simulink model "torque_reflex"  (R2019b)
settings: Solver=ode4  StartTime=0.0  StopTime=inf  FixedStep=BKIN_STEP_TIME  RelTol=1e-3  EnableMultiTasking=on
StartFcn:
  |  warndlg('Dexterit-E models cannot run under simulation. Please compile your model and run it from within Dexterit-E.');set_param(bdroot,'SimulationCommand','stop')
model workspace (MAT data in the model file):
  ACTIVE = 4
  AMPLITUDE = 7
  BASE_STIFFNESS = 12
  BKIN_KINEMATIC_FRAME_SIZE = 400
  BKIN_STEP_TIME = 0.00025
  COLOR_2 = 5
  CONDITION = 3
  DELAY_POST_TRIAL = 4
  DURATION = 5
  E_END_TRIAL = 2
  E_HAND_OUT = 4
  E_NO_EVENT = 0
  E_SHOW_TARGET = 3
  E_SRS_ON = 6
  E_START_TRIAL = 5
  E_TARGET_REACHED = 1
  HAND_OUT_TIME = 6
  IMAGE = 3
  INSERT_OFFSET = 8
  L1_LENGTH = 6
  L1_LINE = 7
  L2_LENGTH = 7
  L2_LINE = 8
  LOAD = 2
  MOVE_THRESHOLD = 10
  MUSCLE = 1
  MUSCLE_LENGTH = 1
  REFLEX = 9
  REFLEX_GAIN = 5
  RESTING_FORCE = 2
  SPEED = 6
  SPRING_X = 1
  SPRING_Y = 2
  SRS_GAIN = 13
  TARGET_1 = 3
  THICKNESS = 4
  V_MAX = 3
  WALL_DAMPING = 11
  WALL_STIFFNESS = 9
  activation = 1
  col_x = 1
  col_y = 2
undefined symbols (not defined in the file or in its folder): slselsubs
libraries: Video x5, simulink x5, xpcutilitieslib x4, KINARM_IO x4, General x3, KINARM_loads x2, KINARM_EP_loads x2, KINARM_general x1, dspstat3 x1
(part 1 of 2)
settings Model: ModifiedComment=chris -- Wed Feb 16 09:18:30 2005 -- Version 1.1384  ModifiedHistory=Feb 16/05 - Add error repeat, add offset ramp  ExtModeArmWhenConnect=off  ExtModeLogAll=off  OrderedModelArguments=off  Creator=Chris Grebeldinger  LastModifiedBy=tinggroup
settings SolverCC: AutoInsertRateTranBlk=on
settings DataIOCC: SaveFormat=Array  SignalLoggingSaveFormat=ModelDataLogs  SaveOutput=off  SaveTime=off  ReturnWorkspaceOutputs=off  SignalLoggingName=sigsOut
settings OptimizationCC: BlockReduction=off  BooleanDataType=off  OptimizeBlockIOStorage=off  BufferReuse=off  GlobalBufferReuse=off  ExpressionFolding=off  ExpressionDepthLimit=2147483647  LocalBlockOutputs=off  InitFltsAndDblsToZero=on  LifeSpan=inf  OptimizeDataStoreBuffers=off  BusAssignmentInplaceUpdate=off
settings DebuggingCC: SaveWithParameterizedLinksMsg=none  UnderspecifiedInitializationDetection=Classic  MergeDetectMultiDrivingBlocksExec=none  SignalResolutionControl=TryResolveAllWithWarning  MultiTaskDSMMsg=warning  FcnCallInpInsideContextMsg=warning  BusObjectLabelMismatch=none  StateNameClashWarn=warning  StrictBusMsg=ErrorOnBusTreatedAsVector  SFUnexpectedBacktrackingDiag=warning  SFNoUnconditionalDefaultTransitionDiag=warning  SFExecutionAtInitializationDiag=none  UnderSpecifiedDimensionMsg=warning  ArithmeticOperatorsInVariantConditions=warning
settings HardwareCC: ProdBitPerPointer=32  ProdBitPerSizeT=32  ProdBitPerPtrDiffT=32  ProdLargestAtomicFloat=None  ProdWordSize=32  ProdLongLongMode=on  ProdHWDeviceType=Generic->32-bit x86 compatible  TargetHWDeviceType=32-bit Generic
settings ModelReferenceCC: PropagateSignalLabelsOutOfModel=off
settings SFSimCC: SimUseLocalCustomCode=off  SimParseCustomCode=off  CustomCodeUndefinedFunction=UseInterfaceOnly
settings RTWCC: Description=Simulink Real-Time  SystemTargetFile=slrt.tlc  TemplateMakefile=slrt_default_tmf  RTWUseLocalCustomCode=off  CustomHeaderCode=#include <stdlib.h>  CodeExecutionProfiling=on  RTWCompilerOptimization=on
settings CodeAppCC: MaxIdLength=63  StateflowObjectComments=on
settings SimulinkRealTimeCC: TargetFcnLib=ansi_tfl_tmw.mat  GeneratePreprocessorConditionals=Disable all  PreserveStateflowLocalDataDimensions=off
settings ConfigComp: CovMetricSettings=dw  CovHtmlReporting=on  CovSaveCumulativeToWorkspaceVar=on  CovSaveSingleToWorkspaceVar=on  CovExternalEMLEnable=off

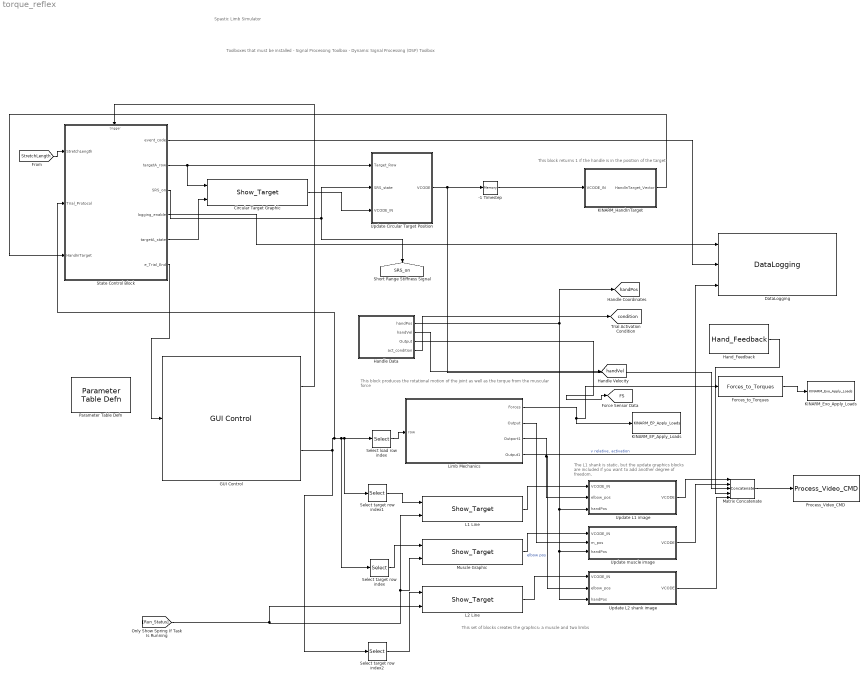
== system torque_reflex ==
  note: The L1 shank is static, but the update graphics blocks are included if you want to add another degree of freedom.
  note: This block returns 1 if the handle is in the position of the target
  note: This set of blocks creates the graphics: a muscle and two limbs
  note: Toolboxes that must be installed
      | - Signal Processing Toolbox
      | - Dynamic Signal Processing (DSP) Toolbox
  note: Spastic Limb Simulator
  note: This block produces the rotational motion of the joint as well as the torque from the muscular force
  "-1 Timestep " : Memory
  Circular Target Graphic : Video/Show_Target  target_type=Circle  num_states=3  attribcol1=[IMAGE IMAGE 0 THICKNESS]  attribcol2=[COLOR_2 COLOR_2 0 THICKNESS]  attribcol3=[COLOR_2 IMAGE 0 THICKNESS]  attribcol4=[0 0 0 0]  attribcol5=[0 0 0 0]  stateindices_padding=[0 0 0 0 0 0 0;0 0 0 0 0 0 0;0 0 0 0 0 0 0;0 0 0 0 0 0 0;0 0 0 0 0 0 0]  source=dialog  opacity=100  target_display=Both subject and operator displays  num_col=4
  DataLogging : General/DataLogging  log_event_codes=on  log_analog_inputs=on  show_time_remaining=off  ecat_include=on
  Forces_to_Torques : KINARM_loads/Forces_to_Torques
  GUI Control : General/GUI Control  task_version=1.0  show_repeat_trial_flag=off  use_custom_tp=off  target_type_str=Circle  Target_Type=1  XYcols=[1 2]  Vcols=3  Lcols=4  indices_padding=[0 0 0 0;0 0 0 0]  target_table_rows=64  load_table_rows=27  tp_table_rows=100
  Hand_Feedback : KINARM_general/Hand_Feedback  feedback_cntl_src=none
  Handle Data : Subsystem
  KINARM_EP_Apply_Loads : KINARM_EP_loads/KINARM_EP_Apply_Loads  up_duration=3000  down_duration=1500  max_force=30
  KINARM_Exo_Apply_Loads : KINARM_loads/KINARM_Exo_Apply_Loads  up_duration=500  down_duration=500  max_torque=7  limit_motors=off
  KINARM_HandInTarget : Subsystem  AncestorBlock=KINARM_general/KINARM_HandInTarget  mask(KINARM_HandInTarget){use_dominant_hand=on, target_type=Circle, num_states=1, attribcol1=[THICKNESS], attribcol2=[0], attribcol3=[0], attribcol4=[0], attribcol5=[0]}
      mask prompts: use_dominant_hand "Use "arm to be assessed"?"; target_type "Type of Target"; num_states "Number of Target States"; attribcol1 "State 1 Target Table Column(s)"; attribcol2 "State 2 Target Table Column(s)"; attribcol3 "State 3 Target Table Column(s)"; attribcol4 "State 4 Target Table Column(s)"; attribcol5 "State 5 Target Table Column(s)"
      mask help: This block returns a vector or array corresponding to the Target_Table rows indicating whether the specified hand is in (=1) or out (=0) of each of the targets.
      mask init:
      | block_path = gcb;  % store block path, as gcb may change with block operations
      | 
      | %%% Get the model's workspace, because it is required to evaluate constants from the Parameter Table Def'n block
      | modelName=bdroot(block_path);
      | modelWorkspace = get_param(modelName, 'ModelWorkspace');
      | 
      | %%% Handle background colours if link status changes.  
      | checkBackgroundColour(block_path, 'KINARM_general');
      | 
      | %%% create the names of the input and output ports to display on the mask
      | % Select only the desired states for output. The output port is also renamed to reflect 
      | % whether the output is a vector (in the case of a single state) or an array (of vectors, 
      | % one for each of multiple states).
      | 
      | numStates = str2double( get_param(block_path, 'num_states') );
      | 
      | if numStates == 1
      | 	set_param([block_path '/Selected States'], 'Value', '[1]');
      | 	outputname = 'HandInTarget_Vector';
      | elseif numStates == 2
      | 	set_param([block_path '/Selected States'], 'Value', '[1,2]');
      | 	outputname = 'HandInTarget_Array';
      | elseif numStates == 3
      | 	set_param([block_path '/Selected States'], 'Value', '[1,2,3]');
      | 	outputname = 'HandInTarget_Array';
      | elseif numStates == 4
      | 	set_param([block_path '/Selected States'], 'Value', '[1,2,3,4]');
      | 	outputname = 'HandInTarget_Array';
      | else
      | 	set_param([block_path '/Selected States'], 'Value', '[1,2,3,4,5]');
      | 	outputname = 'HandInTarget_Array';
      | end
      | output_block=char(find_system(gcb,'LookUnderMasks','all','FollowLinks','on','SearchDepth',1,'BlockType','Outport'));
      | set_param(output_block, 'Name', outputname);
      | 
      | 
      | %%%%%%%%%%%%%%%%%%%%%%%%%%%%%%%%%%%%%%%%%%%%%%%%%%%%%%%%%%%%%
      | %%% Check and format the input strings for the vectors of column entires
      | targetTypeStr=get_param(block_path, 'target_type');
      | 
      | switch targetTypeStr(1:3)
      | 	case 'Cir',		numCol = 1;
      | 	case 'Ell',		numCol = 3;
      |     case 'Rec',		numCol = 3;
      |     case 'Lin',		numCol = 3;
      |     case 'Tri',		numCol = 4;
      | 	otherwise,		numCol = 1;
      | end
      | 
      | for ii = 1:numStates
      | 	variableName = ['attribcol' num2str(ii)];
      | 	attribcoltext = get_param(block_path, variableName);
      | 	attribcoltext = checkUserInputVectorLength(attribcoltext, numCol);
      | 	set_param(block_path, variableName, attribcoltext);
      | end
      | 
      | for ii = 1+numStates:5
      | 	variableName = ['attribcol' num2str(ii)];
      |     if numCol == 1
      |         outstr = '[0]';
      |     else
      |         outstr = mat2str(zeros(1, numCol));
      |     end
      |     set_param(block_path, variableName, outstr);
      | end
      | 
      | %%%%%%%%%%%%%%%%%%%%%%%%%%%%%%%%%%%%%%%%%%%%%%%%%%%%%%%%%%%%%
      | %%% Create the text to show on the mask
      | numStates = str2num(get_param(block_path, 'num_states'));
      | columntext='(columns: ';
      | 
      | for ii = 1:numStates
      | 	variableName = ['attribcol' num2str(ii)];
      | 	attribcolString = get_param(block_path, variableName);
      | 	if isempty(modelWorkspace)
      | 		% if the block is part of a library, then modelWorkspace will be empty and the other code to evaluate attribcolStringEval will fail
      | 		attribcolStringEval = '3';
      | 	else
      | 		[attribcolValue, errorMessage] = BKINevalin(modelWorkspace, attribcolString);
      | 		attribcolStringEval = mat2str( attribcolValue );
      | 	end
      | 	if ii > 1
      | 		columntext = [columntext, '; ', attribcolStringEval];
      | 	else
      | 		columntext = [columntext, attribcolStringEval];
      | 	end
      | end
      | 
      | % Add formatting spaces so that the mask looks nice
      | columntext=strvcat([columntext ')'],' ', ' ');
      mask Help:
      | Used to determine if the hand (fingertip) is in any of the targets in the Target_Table.
      | <P>
      | <B><I>Use of this block requires that the DataLogging block (General library) be set to log KINARM data.</I></B>
      | 
      | <H2>Library </H2>
      | KINARM general
      | 
      | <H2>Description </H2>
      | This block returns a vector or array corresponding to the Target_Table rows indicating whether the specified hand (i.e. fingertip) is in or out of each of the targets.  Each element in the output vector or output array will be either a 0 (hand not in target) or a 1 (hand in target).
      | <P>
      | A vector is returned if only one target state is specified in each target row (see Parameters and Dialog Box), with each index of the vector corresponding to a row in the target table.  An array is returned if more than one target state is specified in a target row, with each row of the array corresponding to a target row and each column corresponding to the nth target state specified in each target row.
      | <P>
      | The output vector or array is typically used by a stateflow chart to affect behavior of the system.  Because this block returns hand-in-target information for all targets in the target table, multiple targets can be monitored at once (i.e. the Stateflow chart could have certain transitions that occur if the hand is in one target and other transitions if it is in a different target).  Likewise, because this block returns hand-in-target information for multiple states of a single target, those multiple states can be monitored simultaneously.
      | <P>
      | Because the KINARM_HandInTarget block returns information for only one hand, two copies of this block are required if information for both hands is desired.
      | <P>
      | 
      | <H2>Parameters and Dialog Box</H2>
      | <B>Use "arm to be assessed"?:</B> this checkbox determines which hand is used by this block. In Dexterit-E the operator selects the "arm to be assessed" using radio buttons.
      | When this box is checked the output of this block is derived from the hand information corresponding to the arm selection made by the operator in Dexterit-E.
      | When this box is unchecked the output of this block is derived from the contralateral arm.
      | (Note: to obtain information about both hands, then 2 separate copies of this block are required - one for each hand.)
      | <P>
      | <B>Type of Target:</B> Enter the type of target specified in the target table:
      | <P>
      | <B>Number of Target States:</B> Enter the number of target states specified in each target row.  Up to four target states are allowed per target row.
      | <P>
      | <B>State <n> Target Table Columns:</B> Enter the columns in the Target Table that specify the relevant target attributes.  Do this for each target state.
      | For a circle, enter the columns corresponding to logical radius (e.g. 4)
      | <BR>For an ellipse, enter the columns corresponding to major radius, minor radius, rotation angle (e.g. [4, 5, 6]).
      | <BR>For a rectangle, enter the columns corresponding to length, height, and rotation angle (e.g. [4, 5, 6]).
      | <BR>For a line, enter the columns corresponding to stroke width, endpoint in x, and endpoint in y (e.g. [3, 4, 5]).
      | <BR>For a triangle, enter the columns corresponding to length, height, peak offset, and rotation angle (e.g. [4, 5, 6, 7]).
      | 
      | <H2>Examples</H2>
      | <B>Example 1.</B>  Suppose a target row will be used to define 1 state for a circle type target and the radius of the visual target is the same radius to be used for determination of hand-in-target.  The related Target Table column is: column 6 = radius.  For this example, "State 1 Target Table Columns" would equal [6].
      | <P>
      | 
      | <B>Example 2.</B>  Suppose a target row will be used to define 1 state for a circle type target, but the radius of the visual target will be different than the radius to be used for determination of hand-in-target.  This option allows independent control over the size of the visual target versus the accuracy needed to be considered "in the target".  The related Target Table columns are: column 6 = radius1 (i.e. radius to target to be drawn); column 7 = radius2 (i.e. radius to be used for hand-in-target) .  For this example, "State 1 Target Table Columns" would equal [7].
      | <P>
      | <B>Example 3.</B>  Suppose a target row will be used to define 2 states for a circle type target, where the radius of the visual target will be a constant, but depending on the state of the system, one of 2 other and different radii will be used for determination of hand-in-target.  The related Target Table columns are: column 6 = radius1 (i.e. radius to target to be drawn); column 7 = radius2 (i.e. radius to be used for hand-in-target for state 1); column 8 = radius3 (i.e. radius to be used for hand-in-target for state 2).  For this example, "State 1 Target Table Columns" would equal [7], while "State 2 Target Table Columns" would equal [8].
      | <P>
      | 
      | <H2>Related Blocks </H2>
      | DataLogging
      mask TypeOptions target_type: Circle | Ellipse | Rectangle | Line | Triangle
      mask Callback target_type:
      | %%%%
      | % Because of bugs iN R2007, R2010a and R2013a (which have been reported to Mathworks), the following code
      | % is required here because in the Initialization Section it will ONLY correctly update those Mask Parameters that are hidden
      | % when the OK button is clicked (NOTE: the initialization code will correctly update all Mask Parameters when the Apply button
      | % is clicked, the bug is that it should also update everything when the OK button is clicked in the absence of an Apply click)
      | %
      | % Adding a set_param call which updates one of the mask parameters will call the initialization code to run, which "avoids"
      | % this bug. This code should be removed once Mathworks has fixed this bug.
      | 
      | temp = get_param(gcb, 'target_type');
      | set_param(gcb, 'target_type', temp);
      mask TypeOptions num_states: 1 | 2 | 3 | 4 | 5
      mask Callback num_states:
      | num_states = str2num(get_param(gcb, 'num_states'));
      | vis = get_param(gcb, 'MaskVisibilities');
      | 
      | % Select only the desired states for output. The output port is also renamed to reflect
      | % whether the output is a vector (in the case of a single state) or an array (of vectors,
      | % one for each of multiple states).
      | output_block=char(find_system(gcb, 'LookUnderMasks', 'all', 'FollowLinks', 'on', 'SearchDepth', 1, 'BlockType', 'Outport'));
      | 
      | if num_states == 1
      | % % % 	set_param([gcb '/Selected States'], 'Value', '[1]');
      | % % % 	set_param(output_block, 'Name', 'HandInTarget_Vector');
      | 	vis{5} = 'off';
      | 	vis{6} = 'off';
      | 	vis{7} = 'off';
      | 	vis{8} = 'off';
      | elseif num_states == 2
      | % % % 	set_param([gcb '/Selected States'], 'Value', '[1,2]');
      | % % % 	set_param(output_block, 'Name', 'HandInTarget_Array');
      | 	vis{5} = 'on';
      | 	vis{6} = 'off';
      | 	vis{7} = 'off';
      | 	vis{8} = 'off';
      | elseif num_states == 3
      | % % % 	set_param([gcb '/Selected States'], 'Value', '[1,2,3]');
      | % % % 	set_param(output_block, 'Name','HandInTarget_Array');
      | 	vis{5} = 'on';
      | 	vis{6} = 'on';
      | 	vis{7} = 'off';
      | 	vis{8} = 'off';
      | elseif num_states == 4
      | % % % 	set_param([gcb '/Selected States'], 'Value', '[1,2,3,4]');
      | % % % 	set_param(output_block, 'Name','HandInTarget_Array');
      | 	vis{5} = 'on';
      | 	vis{6} = 'on';
      | 	vis{7} = 'on';
      | 	vis{8} = 'off';
      | else
      | % % % 	set_param([gcb '/Selected States'], 'Value', '[1,2,3,4,5]');
      | % % % 	set_param(output_block, 'Name', 'HandInTarget_Array');
      | 	vis{5} = 'on';
      | 	vis{6} = 'on';
      | 	vis{7} = 'on';
      | 	vis{8} = 'on';
      | end
      | set_param(gcb, 'MaskVisibilities', vis);
      mask Display:
      | disp(columntext);
      | port_label('output',1,outputname);
  L1 Line : Video/Show_Target  target_type=Line  num_states=1  attribcol1=[IMAGE IMAGE THICKNESS col_x col_x]  attribcol2=[0 0 0 0 0]  attribcol3=[0 0 0 0 0]  attribcol4=[0 0 0 0 0]  attribcol5=[0 0 0 0 0]  stateindices_padding=[0 0 0 0 0 0;0 0 0 0 0 0;0 0 0 0 0 0;0 0 0 0 0 0;0 0 0 0 0 0]  source=dialog  opacity=100  target_display=Both subject and operator displays  num_col=5
  L2 Line : Video/Show_Target  target_type=Line  num_states=1  attribcol1=[IMAGE IMAGE THICKNESS col_x col_y]  attribcol2=[0 0 0 0 0]  attribcol3=[0 0 0 0 0]  attribcol4=[0 0 0 0 0]  attribcol5=[0 0 0 0 0]  stateindices_padding=[0 0 0 0 0 0;0 0 0 0 0 0;0 0 0 0 0 0;0 0 0 0 0 0;0 0 0 0 0 0]  source=dialog  opacity=100  target_display=Both subject and operator displays  num_col=5
  "Limb Mechanics " : Subsystem  mask(Constant_Loads(Bimanual_Spring)){loadcol=[1   2   3   4   5   6   7   8   9  10  11  12  13]}
      mask prompts: loadcol "Load Table columns [A B C]"
      mask help:
      | The Hill Model creates constant loads on the KINARM in a global cartesian space.
      |
      | The force produced is modeled by a Hill-type model of Force-Length and Force-Velocity Relationships.
      |
      | Loading parameters come from Load Table columns [A B C].
      |
      | Column A: Rest Length "t0" (m)
      | Column B: Rest Tension (N)
      | Column C: Maximum Stretch Velocity (Kg/s)
      | (Enter 0 to not use a value.  Defaults are 0m, 0 N/m and 10 (t0/s))
      mask init:
      | columntext = strvcat('(columns)', get_param(gcb, 'loadcol'));
      | 
      | input_block = find_system(gcb,'LookUnderMasks','all','FollowLinks','on','SearchDepth',1,'BlockType','Inport');
      | output_block = find_system(gcb,'LookUnderMasks','all','FollowLinks','on','SearchDepth',1,'BlockType','Outport');
      | 
      | inputname1=get_param(char(input_block(1)),'Name');
      | outputname1 = get_param(char(output_block(1)),'Name');
      mask Callback loadcol:
      | loadcol=[str2num(get_param(gcb, 'loadcol')) 0 0 0];
      | set_param(gcb, 'loadcol', ['[' num2str(loadcol(1:13)) ']']);
      mask Display:
      | disp(columntext)
      | port_label('output',1,outputname1)
      | port_label('input',1, inputname1)
  Matrix Concatenate : Concatenate  NumInputs=5  Mode=Multidimensional array
  Muscle Graphic : Video/Show_Target  target_type=Line  num_states=1  attribcol1=[IMAGE IMAGE THICKNESS col_x col_x]  attribcol2=[0 0 0 0 0]  attribcol3=[0 0 0 0 0]  attribcol4=[0 0 0 0 0]  attribcol5=[0 0 0 0 0]  stateindices_padding=[0 0 0 0 0 0;0 0 0 0 0 0;0 0 0 0 0 0;0 0 0 0 0 0;0 0 0 0 0 0]  source=dialog  opacity=100  target_display=Both subject and operator displays  num_col=5
  Parameter Table Defn : General/Parameter Table Defn  ShowInLibBrowser=0
  Process_Video_CMD : Video/Process_Video_CMD  video_delay=0
  Select load row index : Selector  IndexOptions=Index vector (dialog)  Indices=LOAD  OutputSizes=slselsubs([(-2),(-2)],1)
  Select target row index : Selector  IndexOptions=Index vector (dialog)  Indices=MUSCLE  OutputSizes=slselsubs([(-2),(-2)],1)
  Select target row index1 : Selector  IndexOptions=Index vector (dialog)  Indices=L1_LINE  OutputSizes=slselsubs([(-2),(-2)],1)
  Select target row index2 : Selector  IndexOptions=Index vector (dialog)  Indices=L2_LINE  OutputSizes=slselsubs([(-2),(-2)],1)
  State Control Block : Stateflow chart  TreatAsAtomicUnit=on
  Update Circular Target Position : Subsystem
  Update L1 image : MATLAB Function  TreatAsAtomicUnit=on
  Update L2 shank image : MATLAB Function  TreatAsAtomicUnit=on
  Update muscle image : MATLAB Function  TreatAsAtomicUnit=on
  tag scope: FS=global, SRS_on=global, condition=global, handPos=global, handVel=global
  wires:
  "Limb Mechanics "/4(Output1) -> DataLogging/3  "v relative, activation"
  Handle Data/3(Output) -> [FS]
  [Run_Status] -> Muscle Graphic/2, L1 Line/2, L2 Line/2
  Select load row index/1 -> "Limb Mechanics "/1(row)
  Hand_Feedback/1 -> Matrix Concatenate/4
  Handle Data/1(handPos) -> [handPos], Update muscle image/3(handPos), Update L2 shank image/3(handPos), Update L1 image/3(handPos)
  Handle Data/2(handVel) -> [handVel]
  Select target row index/1 -> Muscle Graphic/1
  "Limb Mechanics "/2(Output) -> Update muscle image/2(m_pos)
  Update L1 image/1(VCODE) -> Matrix Concatenate/1
  "-1 Timestep "/1 -> KINARM_HandInTarget/1("VCODE_IN ")
  L1 Line/1 -> Update L1 image/1(VCODE_IN)
  KINARM_HandInTarget/1(HandInTarget_Vector) -> State Control Block/3(HandInTarget)
  Select target row index2/1 -> L2 Line/1
  Select target row index1/1 -> L1 Line/1
  "Limb Mechanics "/3(Outport1) -> Update L1 image/2(elbow_pos), Update L2 shank image/2(elbow_pos)  "elbow pos"
  Forces_to_Torques/1 -> KINARM_Exo_Apply_Loads/1
  State Control Block/6(e_Trial_End) -> GUI Control/1
  State Control Block/4(logging_enable) -> DataLogging/1
  Circular Target Graphic/1 -> Update Circular Target Position/3("VCODE_IN ")
  State Control Block/1(event_code) -> DataLogging/2
  "Limb Mechanics "/1(Forces) -> KINARM_EP_Apply_Loads/1, Forces_to_Torques/1
  Muscle Graphic/1 -> Update muscle image/1(VCODE_IN)
  L2 Line/1 -> Update L2 shank image/1(VCODE_IN)
  Update muscle image/1(VCODE) -> Matrix Concatenate/2
  Matrix Concatenate/1 -> Process_Video_CMD/1
  GUI Control/1 -> State Control Block/Trigger
  Update L2 shank image/1(VCODE) -> Matrix Concatenate/5
  State Control Block/2(targetA_row) -> Circular Target Graphic/1, Update Circular Target Position/1(Target_Row)
  GUI Control/2 -> Select target row index/1, Select load row index/1, Select target row index1/1, State Control Block/2(Trial_Protocol), Select target row index2/1
  Update Circular Target Position/1(VCODE) -> "-1 Timestep "/1, Matrix Concatenate/3
  Handle Data/4(act_condition) -> [condition]
  [StretchLength] -> State Control Block/1(StretchLength)
  State Control Block/5(targetA_state) -> Circular Target Graphic/2
  State Control Block/3(SRS_on) -> [SRS_on], Update Circular Target Position/2(SRS_state)

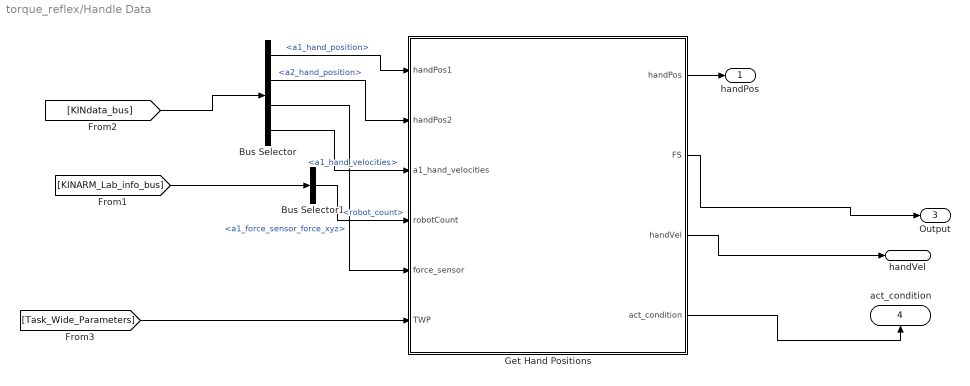
== system torque_reflex/Handle Data ==
  Bus Selector : BusSelector  OutputSignals=Robot1.a1_hand_position,Robot2.a2_hand_position,Robot1.a1_force_sensor_force_xyz,Robot1.a1_hand_velocities
  Bus Selector1 : BusSelector  OutputSignals=robot_count
  Get Hand Positions : MATLAB Function  TreatAsAtomicUnit=on
  handPos : Outport
  handVel : Outport  Port=2
  Output : Outport  Port=3
  act_condition : Outport  Port=4
  wires:
  Get Hand Positions/2(FS) -> Output/1
  Bus Selector/3 -> Get Hand Positions/5(force_sensor)  "<a1_force_sensor_force_xyz>"
  Bus Selector1/1 -> Get Hand Positions/4(robotCount)  "<robot_count>"
  Bus Selector/1 -> Get Hand Positions/1(handPos1)  "<a1_hand_position>"
  Bus Selector/2 -> Get Hand Positions/2(handPos2)  "<a2_hand_position>"
  [KINdata_bus] -> Bus Selector/1
  [KINARM_Lab_info_bus] -> Bus Selector1/1
  [Task_Wide_Parameters] -> Get Hand Positions/6(TWP)
  Get Hand Positions/1(handPos) -> handPos/1
  Bus Selector/4 -> Get Hand Positions/3(a1_hand_velocities)  "<a1_hand_velocities>"
  Get Hand Positions/3(handVel) -> handVel/1
  Get Hand Positions/4(act_condition) -> act_condition/1

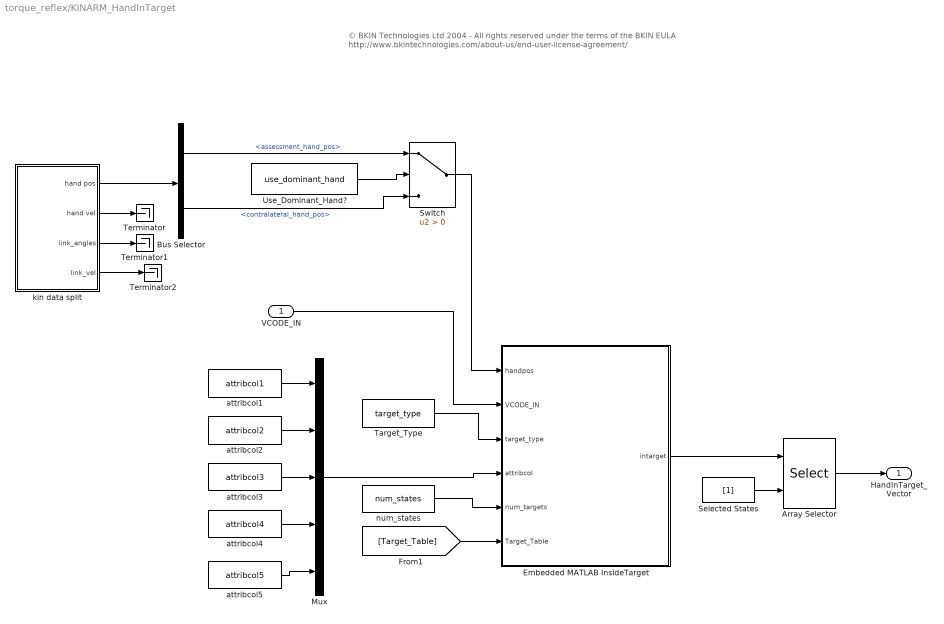
== system torque_reflex/KINARM_HandInTarget ==
  note: © BKIN Technologies Ltd 2004  - All rights reserved under the terms of the BKIN EULA
      | http://www.bkintechnologies.com/about-us/end-user-license-agreement/
  "VCODE_IN " : Inport
  Array Selector : Selector  NumberOfDimensions=2  InputPortWidth=3  IndexOptions=Select all,Index vector (port)  Indices=-1,1  OutputSizes=slselsubs([(-2),(-2)],1),slselsubs([(-2),(-2)],2)
  Bus Selector : BusSelector  OutputSignals=assessment_hand_pos,contralateral_hand_pos
  Embedded MATLAB InsideTarget : MATLAB Function  TreatAsAtomicUnit=on
      settings: RTWSystemCode=Nonreusable function  RTWFileNameOpts=Use function name
  Mux : Mux  Inputs=5
  Selected States : Constant  Value=[1]
  Switch : Switch  Criteria=u2 > Threshold
  Target_Type : Constant  Value=target_type
  Terminator : Terminator
  Terminator1 : Terminator
  Terminator2 : Terminator
  Use_Dominant_Hand? : Constant  Value=use_dominant_hand
  attribcol1 : Constant  Value=attribcol1
  attribcol2 : Constant  Value=attribcol2
  attribcol3 : Constant  Value=attribcol3
  attribcol4 : Constant  Value=attribcol4
  attribcol5 : Constant  Value=attribcol5
  kin data split : Subsystem
  num_states : Constant  Value=num_states
  HandInTarget_Vector : Outport
  wires:
  Selected States/1 -> Array Selector/2
  num_states/1 -> Embedded MATLAB InsideTarget/5(num_targets)
  Mux/1 -> Embedded MATLAB InsideTarget/4(attribcol)
  attribcol4/1 -> Mux/4
  attribcol3/1 -> Mux/3
  attribcol2/1 -> Mux/2
  attribcol1/1 -> Mux/1
  Target_Type/1 -> Embedded MATLAB InsideTarget/3(target_type)
  Array Selector/1 -> HandInTarget_Vector/1
  [Target_Table] -> Embedded MATLAB InsideTarget/6(Target_Table)
  Embedded MATLAB InsideTarget/1(intarget) -> Array Selector/1
  attribcol5/1 -> Mux/5
  kin data split/1(hand pos) -> Bus Selector/1
  Use_Dominant_Hand?/1 -> Switch/2
  Bus Selector/1 -> Switch/1  "<assessment_hand_pos>"
  Bus Selector/2 -> Switch/3  "<contralateral_hand_pos>"
  kin data split/2(hand vel) -> Terminator/1
  kin data split/3(link_angles) -> Terminator1/1
  Switch/1 -> Embedded MATLAB InsideTarget/1(handpos)
  "VCODE_IN "/1 -> Embedded MATLAB InsideTarget/2(VCODE_IN)
  kin data split/4(link_vel) -> Terminator2/1

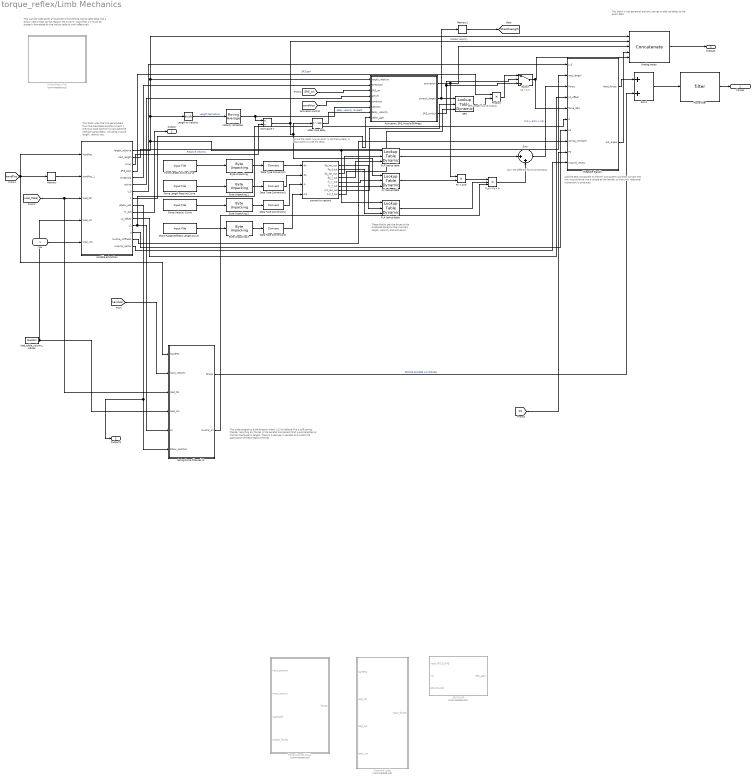
== system torque_reflex/Limb Mechanics  ==
  note: Sum the different force components
  note: Add the SRS component to the Hill Component and then convert the raw muscle force into a torque at the handle, so that only rotational movement is produced
  note: Since the robot runs at 4kHz, a 120 frame delay is equivalent to a 30 ms delay
  note: This block uses the trial parameters from the load table and the current + previous hand position to calculate the relevant parameters, including muscle length, velocity etc.
  note: These blocks get the forces to be produced based on the muscle's length, velocity and activation.
  note: This code programs a the forearm shank (L2) to behave like a stiff spring, thereby resisting any forces in the parallel component that would lengthen or shorten the forearm length. There is a damper in parallel to smooth the application of these reactive forces
  note: This block is not essential and only serves to add variables to the exam data
  note: This sample code gives an example of converting lookup table data into a binary vector that can be read by the KinArm. Input files 1-4 must be properly formatted for the lookup table to work effectively
  row : Inport
  "Activation, SRS, Muscle Stiffness" : MATLAB Function  TreatAsAtomicUnit=on
  Analog Inputs : Concatenate  NumInputs=5  Mode=Multidimensional array  ConcatenateDimension=2
  Byte Unpacking {,1..3} (4 alike) : xpcutilitieslib/Byte Unpacking   MaskUnpackedDataTypes={'single'}  MaskUnpackedDataSizes={2}  MaskAlignment=1
      settings: SourceProductName=Simulink Real-Time  SourceProductBaseCode=XP
  Constant Loads : MATLAB Function  Commented=on  TreatAsAtomicUnit=on
  Data Type Conversion{,1..3} (4 alike) : DataTypeConversion
  FLA * FV * A : Product  Inputs=3
  FLA lookup table : simulink/Lookup Tables/Lookup Table Dynamic  LookUpMeth=Interpolation-Use End Values  OutDataType=fixdt('double')  OutScaling=[]  OutputDataTypeScalingMode=Specify via dialog  OutDataTypeStr=double  DoSatur=off
      settings: SourceProductName=Simulink
  FLP lookup table : simulink/Lookup Tables/Lookup Table Dynamic  LookUpMeth=Interpolation-Use End Values  OutDataType=fixdt('double')  OutScaling=[]  OutputDataTypeScalingMode=Specify via dialog  OutDataTypeStr=double  DoSatur=off
      settings: SourceProductName=Simulink
  FV * ACT : Product
  "FV lookup table " : simulink/Lookup Tables/Lookup Table Dynamic  LookUpMeth=Interpolation-Use End Values  OutDataType=fixdt('double')  OutScaling=[]  OutputDataTypeScalingMode=Specify via dialog  OutDataTypeStr=double  DoSatur=off
      settings: SourceProductName=Simulink
  Force Channel WALL : MATLAB Function  Commented=on  TreatAsAtomicUnit=on
  Force Length Active Curve : KINARM_IO/Input File  filenameid=1  dexname='Force Length'  filename='kinarm\1.dat'  dataSize=8  bufSize=2048  readSize=512  EOFOption=Hold last output  sampTime=0.001  show2ports=off
  Force Length Passive Curve : KINARM_IO/Input File  filenameid=2  dexname='Force Length Passive'  filename='kinarm\2.dat'  dataSize=8  bufSize=2048  readSize=512  EOFOption=Hold last output  sampTime=0.001  show2ports=off
  "Force Velocity Curve " : KINARM_IO/Input File  filenameid=3  dexname='Force Velocity'  filename='kinarm\3.dat'  dataSize=8  bufSize=2048  readSize=512  EOFOption=Hold last output  sampTime=0.001  show2ports=off
  Force filter : KINARM_EP_loads/Velocity_Loads_EP/filter  SystemSampleTime=-1  Latency=0  AutoFrameSizeCalculation=off
  Integrate Signals : MATLAB Function  TreatAsAtomicUnit=on
  Length to Velocity : Derivative
  Memory : Memory
  Memory1 : Memory
  Normalize V : Product  Inputs=*/
  Product : Product
  SRS : simulink/Lookup Tables/Lookup Table Dynamic  LookUpMeth=Interpolation-Use End Values  OutDataType=fixdt('double')  OutScaling=[]  OutputDataTypeScalingMode=Specify via dialog  OutDataTypeStr=double  DoSatur=off
      settings: SourceProductName=Simulink
  SRS RAMP : Subsystem  Commented=on  TreatAsAtomicUnit=on
  Short Range Stiffness Length Curve : KINARM_IO/Input File  filenameid=4  dexname='Short Range Stiffness'  filename='kinarm\4.dat'  dataSize=8  bufSize=2048  readSize=512  EOFOption=Seek to beginning  sampTime=0.001  show2ports=off
  Spring Force Channel L2 : MATLAB Function  TreatAsAtomicUnit=on
  Sum : Sum  Inputs=|++
  Sum1 : Sum
  Switch : Switch  Criteria=u2 ~= 0
  Velocity Smoother : dspstat3/Moving Average  Method=Sliding window  ForgettingFactorPort=off  SpecifyWindowLength=on  WindowLength=4  ForgettingFactor=0.9  SimulateUsing=Code generation
  Write Binary File : MATLAB Function  Commented=on  TreatAsAtomicUnit=on
  convert to vectors : MATLAB Function  TreatAsAtomicUnit=on
  load_table_column_indices : Constant  Value=loadcol
  reflex loop delay : Delay  DelayLength=120
  variable extraction : MATLAB Function  TreatAsAtomicUnit=on
  Forces : Outport
  Output : Outport  Port=2
  Outport1 : Outport  Port=3
  Output1 : Outport  Port=4
  tag scope: StretchLength=global
  wires:
  Switch/1 -> Integrate Signals/5(force_SRS), Analog Inputs/5
  convert to vectors/4(flp_f_out) -> FLP lookup table/3
  variable extraction/8(k) -> "Activation, SRS, Muscle Stiffness"/8(reflex_gain)
  Sum/1 -> Integrate Signals/3(Force)  "FLP + a(FV + FA)"
  [handVel] -> Spring Force Channel L2/2(hand_velocity)
  variable extraction/2(rest_length) -> Integrate Signals/2(rest_length)
  SRS/1 -> Product/2  "SRS Length Curve Output"
  Byte Unpacking 2/1 -> Data Type Conversion2/1
  "Force Velocity Curve "/1 -> Byte Unpacking 2/1
  row/1 -> variable extraction/5(load_row)
  FLA * FV * A/1 -> Sum/2
  Normalize V/1 -> "FV lookup table "/1, reflex loop delay/1, Analog Inputs/2  "Scaled Velocity"
  variable extraction/6(active) -> "Activation, SRS, Muscle Stiffness"/4(active)
  "FV lookup table "/1 -> FV * ACT/2
  Integrate Signals/2(out_angle) -> Analog Inputs/4
  variable extraction/4(SRS_gain) -> Product/1  "SRS gain"
  Product/1 -> Switch/1
  Data Type Conversion3/1 -> convert to vectors/4(srs)
  [handPos] -> Spring Force Channel L2/1(handPos), variable extraction/1(handPos), Memory/1
  Sum1/1 -> Force filter/1
  Spring Force Channel L2/2(muscle_on) -> FLA * FV * A/3
  variable extraction/13(d) -> Integrate Signals/7(L2)
  [Load_Table] -> variable extraction/3(load_tbl), Spring Force Channel L2/3(load_tbl)
  FLA lookup table/1 -> FLA * FV * A/2
  variable extraction/15(muscle_vector) -> Integrate Signals/10(muscle_vector)
  variable extraction/3(Vmax) -> Normalize V/2  "Relative Velocity"
  convert to vectors/7(srs_len_out) -> SRS/2
  Force Length Active Curve/1 -> "Byte Unpacking "/1
  [SRS_on] -> "Activation, SRS, Muscle Stiffness"/3(SRS_on)
  [FS] -> Integrate Signals/9(FS)
  variable extraction/10(m_pos) -> Output/1
  "Activation, SRS, Muscle Stiffness"/2(stretch_length) -> Memory1/1, SRS/1
  [condition] -> "Activation, SRS, Muscle Stiffness"/5(condition)
  variable extraction/11(L2_offset) -> Integrate Signals/4(L2_offset)
  variable extraction/14(muscle_stiffness) -> Integrate Signals/8(spring_constant)
  convert to vectors/2(fla_f_out) -> FLA lookup table/3
  Short Range Stiffness Length Curve/1 -> Byte Unpacking 3/1
  Analog Inputs/1 -> Output1/1
  convert to vectors/8(srs_f_out) -> SRS/3
  variable extraction/1(length_relative) -> FLA lookup table/1, FLP lookup table/1, Analog Inputs/1, "Activation, SRS, Muscle Stiffness"/1(length_relative), Length to Velocity/1
  Byte Unpacking 3/1 -> Data Type Conversion3/1
  Byte Unpacking 1/1 -> Data Type Conversion1/1
  convert to vectors/6(fv_f_out) -> "FV lookup table "/3
  "Byte Unpacking "/1 -> Data Type Conversion/1
  FLP lookup table/1 -> Sum/1
  variable extraction/5(threshold) -> "Activation, SRS, Muscle Stiffness"/2(threshold)
  convert to vectors/5(fv_v_out) -> "FV lookup table "/2
  Force Length Passive Curve/1 -> Byte Unpacking 1/1
  Force filter/1 -> Forces/1
  Data Type Conversion1/1 -> convert to vectors/2(flp)
  Data Type Conversion/1 -> convert to vectors/1(fla)
  Integrate Signals/1(hand_forces) -> Sum1/1
  variable extraction/7(t_0) -> Integrate Signals/1(t_0)
  Memory/1 -> variable extraction/2(handPos_1)
  convert to vectors/1(fla_len_out) -> FLA lookup table/2
  Length to Velocity/1 -> Velocity Smoother/1  "Length Derivative"
  convert to vectors/3(flp_len_out) -> FLP lookup table/2
  Data Type Conversion2/1 -> convert to vectors/3(fv)
  reflex loop delay/1 -> "Activation, SRS, Muscle Stiffness"/7(delay_velocity)  "delay velocity (scaled)"
  FV * ACT/1 -> FLA * FV * A/1
  variable extraction/12(L2) -> Integrate Signals/6(d), Spring Force Channel L2/5(L2)
  Memory1/1 -> [StretchLength]
  Spring Force Channel L2/1(forces) -> Sum1/2  "SPRING DAMPER L2 FORCES"
  "Activation, SRS, Muscle Stiffness"/3(SRS_switch) -> Switch/2, Switch/3
  Velocity Smoother/1 -> Normalize V/1, "Activation, SRS, Muscle Stiffness"/6(velocity)
  load_table_column_indices/1 -> Spring Force Channel L2/4(load_col), variable extraction/4(load_col)
  variable extraction/9(elbow_pos) -> Spring Force Channel L2/6(elbow_position), Outport1/1
  "Activation, SRS, Muscle Stiffness"/1(activation) -> Analog Inputs/3, FV * ACT/1

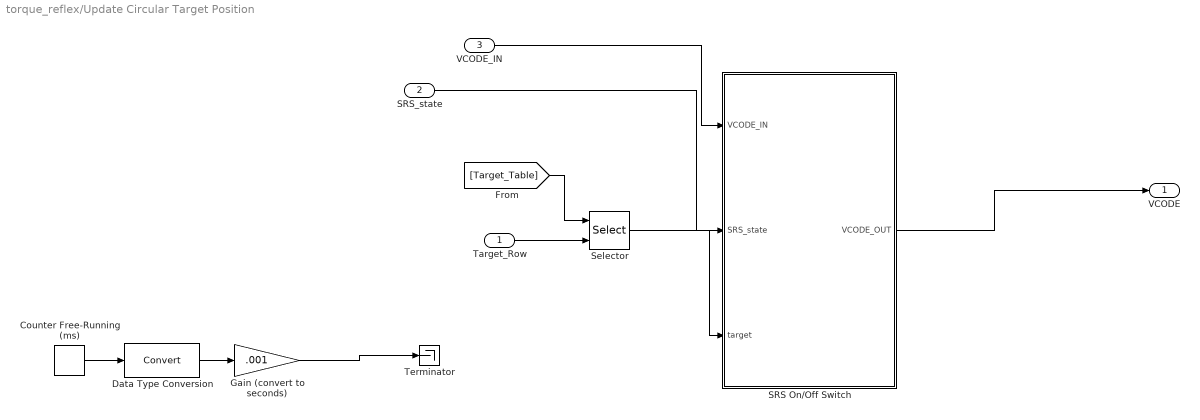
== system torque_reflex/Update Circular Target Position ==
  Target_Row : Inport
  SRS_state : Inport  Port=2
  "VCODE_IN " : Inport  Port=3
  Counter Free-Running (ms) : simulink/Sources/Counter Free-Running  NumBits=32  tsamp=.001
  Data Type Conversion : DataTypeConversion
  Gain (convert to seconds) : Gain  Gain=.001
  SRS On/Off Switch : MATLAB Function  TreatAsAtomicUnit=on
  Selector : Selector  NumberOfDimensions=2  InputPortWidth=3  IndexOptions=Index vector (port),Select all  Indices=1,-1  OutputSizes=1
  Terminator : Terminator
  VCODE : Outport
  wires:
  "VCODE_IN "/1 -> SRS On/Off Switch/1(VCODE_IN)
  SRS On/Off Switch/1(VCODE_OUT) -> VCODE/1
  Target_Row/1 -> Selector/2
  [Target_Table] -> Selector/1
  Selector/1 -> SRS On/Off Switch/3(target)
  Counter Free-Running (ms)/1 -> Data Type Conversion/1
  Data Type Conversion/1 -> Gain (convert to seconds)/1
  Gain (convert to seconds)/1 -> Terminator/1
  SRS_state/1 -> SRS On/Off Switch/2(SRS_state)

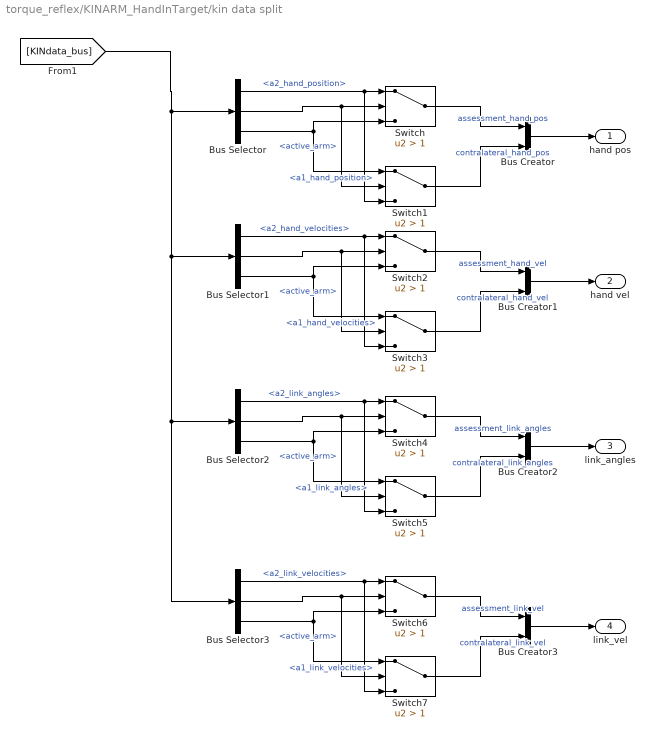
== system torque_reflex/KINARM_HandInTarget/kin data split ==
  Bus Creator{,1..3} (4 alike) : BusCreator  Inputs=2
  Bus Selector : BusSelector  OutputSignals=Robot2.a2_hand_position,KINDataGeneral.active_arm,Robot1.a1_hand_position
  Bus Selector1 : BusSelector  OutputSignals=Robot2.a2_hand_velocities,KINDataGeneral.active_arm,Robot1.a1_hand_velocities
  Bus Selector2 : BusSelector  OutputSignals=Robot2.a2_link_angles,KINDataGeneral.active_arm,Robot1.a1_link_angles
  Bus Selector3 : BusSelector  OutputSignals=Robot2.a2_link_velocities,KINDataGeneral.active_arm,Robot1.a1_link_velocities
  Switch{,1..7} (8 alike) : Switch  Criteria=u2 > Threshold  Threshold=1
  hand pos : Outport
  hand vel : Outport  Port=2
  link_angles : Outport  Port=3
  link_vel : Outport  Port=4
  wires:
  Bus Selector/1 -> Switch1/3, Switch/1  "<a2_hand_position>"
  Switch/1 -> Bus Creator/1  "assessment_hand_pos"
  Switch1/1 -> Bus Creator/2  "contralateral_hand_pos"
  Bus Creator/1 -> hand pos/1
  Bus Selector/3 -> Switch1/1, Switch/3  "<a1_hand_position>"
  Bus Selector/2 -> Switch1/2, Switch/2  "<active_arm>"
  Bus Selector1/1 -> Switch3/3, Switch2/1  "<a2_hand_velocities>"
  Switch2/1 -> Bus Creator1/1  "assessment_hand_vel"
  Switch3/1 -> Bus Creator1/2  "contralateral_hand_vel"
  Bus Creator1/1 -> hand vel/1
  Bus Selector1/3 -> Switch3/1, Switch2/3  "<a1_hand_velocities>"
  Bus Selector1/2 -> Switch3/2, Switch2/2  "<active_arm>"
  Bus Selector2/1 -> Switch5/3, Switch4/1  "<a2_link_angles>"
  Switch4/1 -> Bus Creator2/1  "assessment_link_angles"
  Switch5/1 -> Bus Creator2/2  "contralateral_link_angles"
  Bus Creator2/1 -> link_angles/1
  Bus Selector2/3 -> Switch5/1, Switch4/3  "<a1_link_angles>"
  Bus Selector2/2 -> Switch5/2, Switch4/2  "<active_arm>"
  Bus Selector3/1 -> Switch7/3, Switch6/1  "<a2_link_velocities>"
  Switch6/1 -> Bus Creator3/1  "assessment_link_vel"
  Switch7/1 -> Bus Creator3/2  "contralateral_link_vel"
  Bus Creator3/1 -> link_vel/1
  [KINdata_bus] -> Bus Selector3/1, Bus Selector2/1, Bus Selector1/1, Bus Selector/1
  Bus Selector3/3 -> Switch7/1, Switch6/3  "<a1_link_velocities>"
  Bus Selector3/2 -> Switch7/2, Switch6/2  "<active_arm>"

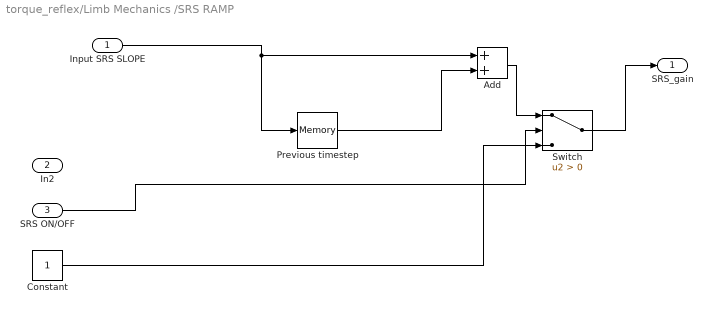
== system torque_reflex/Limb Mechanics /SRS RAMP ==
  Input SRS SLOPE : Inport
  In2 : Inport  Port=2
  SRS ON/OFF : Inport  Port=3
  Add : Sum
  Constant : Constant
  Previous timestep : Memory  InitialCondition=1
  Switch : Switch  Criteria=u2 > Threshold
  "SRS_gain " : Outport
  wires:
  SRS ON/OFF/1 -> Switch/2
  Input SRS SLOPE/1 -> Previous timestep/1, Add/1
  Previous timestep/1 -> Add/2
  Add/1 -> Switch/1
  Constant/1 -> Switch/3
  Switch/1 -> "SRS_gain "/1

== matlab function torque_reflex/Update muscle image ==
  data: VCODE_IN input; m_pos input; VCODE output; handPos input
function VCODE = update_position(VCODE_IN, m_pos, handPos)

% This function takes a VCODE that draws a line and updates the starting and end-point of the line
% In this particular instance however, the 'line' will have a graphic pasted over it.

VCODE = VCODE_IN;

handPos1 = handPos(1, :);  %EP Hand position
handPos2 = handPos(2, :); %origin 

% update VCODE starting and endpoint positions (i.e. assumes that VCODE is for a line).
VCODE(3:4) = m_pos; %start of the line Vcode (x,y coordinates)
VCODE(10:11) = handPos2 - m_pos;  %end of the line
%set the relative position from one hand to the other

== matlab function torque_reflex/Handle Data/Get Hand Positions ==
  data: handPos output; handPos1 input; handPos2 input; a1_hand_velocities input; robotCount input; force_sensor input; TWP input; SPRING_X parameter; SPRING_Y parameter; FS output; handVel output; act_condition output
function [handPos, FS, handVel, act_condition] = get_hand_position(handPos1, handPos2, a1_hand_velocities, robotCount, force_sensor, TWP, SPRING_X, SPRING_Y)

% For bilateral Kinarms, draw the spring between the two hands/handles.
% For unilateral Kinarms, grab the origin of the spring from the Task Wide Parameters.

if robotCount == 1
	handPos2 = [TWP(SPRING_X), TWP(SPRING_Y)];
end

act_condition = TWP(3);



handVel = a1_hand_velocities;

handPos = [handPos1; handPos2];
FS = force_sensor;



end

== matlab function torque_reflex/Limb Mechanics /variable extraction ==
  settings: fimath=|
      | fimath(...
      | 'RoundMode', 'floor',...
      | 'OverflowMode', 'wrap',...
      | 'ProductMode', 'KeepLSB', 'ProductWordLength', 32,...
      | 'SumMode', 'KeepLSB', 'SumWordLength', 32,...
      | 'CastBeforeSum', false)
  data: handPos input; handPos_1 input; load_tbl input; load_col input; length_relative output; rest_length output; Vmax output; SRS_gain output; threshold output; active output; load_row input; t_0 output; k output; elbow_pos output; m_pos output; L2_offset output; L2 output; d output; muscle_stiffness output; muscle_vector output
function [length_relative,rest_length, Vmax, SRS_gain, threshold, active, t_0, k,elbow_pos,m_pos, L2_offset, L2, d,  muscle_stiffness, muscle_vector] = length_velocity(handPos, handPos_1, load_tbl, load_col, load_row)

%initialize default values for any parameters that are not specified in the
%load table!
rest_length = 0.2;				%  default rest length (m)
t_0 = 0;			% resting tension in muscle (N)
muscle_stiffness = 1; %parallel spring stiffness = 1!
Vmax = 10;           %default Vmax in resting lengths per second!
k = 0; %default have no reflex gain
threshold = 0.03; %default threshold
active = 0;
L1 = 0.313; %these should get replaced by the load table values
L2 = 0.313;
d = 0.08; %proportion of length down the forearm of muscle insertion point

SRS_gain = 1;

hand1_pos = handPos(1, :);% instantaneous hand position (x,y)
hand2_pos = handPos(2, :); % instantaneous hand position (x, y)

if load_row > 0 && load_row <= size(load_tbl,1) 
    %muscle resting length l0
    if load_col(1) > 0
        rest_length = abs(load_tbl( load_row, load_col(1)));
    end
    if load_col(2) > 0 %resting tension
        t_0 = load_tbl( load_row, load_col(2)); 
        %Safety limit to keep the KINARM from going unstable, max t0 of 100N
        if t_0 > 100
            t_0 = 100;
        end
    end
    if load_col(3) > 0 
        Vmax = load_tbl(load_row, load_col(3));
        %Vmax is resting lengths per second, usually 10-15
    end
    if load_col(4) > 0
        active = load_tbl(load_row, load_col(4));
    end
    if load_col(5) > 0 %k = reflex gain
        k = load_tbl(load_row, load_col(5));
    end
    if load_col(6) > 0 % L1 length
        L1 = load_tbl(load_row, load_col(6));
    end
    if load_col(7) > 0
        L2 = load_tbl(load_row,load_col(7));
    end 
    if load_col(8) > 0 %d is the distance from joint to muscle insertion along L2 shank
        d = load_tbl(load_row, load_col(8));
    end
    %skip load_col(9) (spring strength). This is handled in another block. 
    if load_col(10) > 0 % resting/moving velocity threshold
        threshold = load_tbl(load_row, load_col(10));
    end
    if load_col(12) > 0
        muscle_stiffness = load_tbl(load_row, load_col(12));
    end
    if load_col(13) > 0
        SRS_gain = load_tbl(load_row, load_col(13));
    end
end
%% now use L1, L2, and L3 to get the muscle length

elbow_pos = hand2_pos - [0, L1]; % elbow is vertically positioned!
%L3_vec = hand2_pos - hand1_pos; %L3_vec is the vector b/w origin and EP
%L3 = sqrt( sum( L3_vec.^2 ) ); %L3 is the size of L3_vec, for use in trigonometric calculations

L2_offset = hand1_pos - elbow_pos; %offset from elbow to hand position for line starting from elbow pos
L2_size = sqrt(sum(L2_offset.^2)); %instantaneous L2_size (should be == L2, because we are trying to fix the position!)

new_mag = d/L2_size;

m_offset = new_mag * L2_offset; %vector from elbow of magnitude d (offset from elbow)

%also calculate the insertion point p(x,y) to update the VR image
m_pos = elbow_pos + m_offset;

muscle_vector = hand2_pos - m_pos; %origin minus muscle position gives muscle to origin vector. 
muscle_length = sqrt(sum(muscle_vector.^2));

length_relative = muscle_length/rest_length; %muscle length over resting tension;


hand1_pos_old = handPos_1(1,:);
hand2_pos_old = handPos_1(2,:);


L2_offset_2 = hand1_pos_old - elbow_pos; %offset from elbow to hand position for line starting from elbow pos
L2_size = sqrt(sum(L2_offset_2.^2));


new_mag = d/L2_size;

m_offset = new_mag * L2_offset; %vector from elbow of magnitude d (offset from elbow)

m_pos2 = elbow_pos + m_offset;

muscle_vector_prev = hand2_pos_old - m_pos2;

muscle_length_prev = sqrt(sum(muscle_vector_prev.^2));

diff = muscle_length - muscle_length_prev;

% theta_diff = theta2 - theta1;

timestep = 0.00025; % 4 kHz ---> 1 frame = 1/4000 seconds or 1 msec

muscle_velocity = diff/timestep; %instantaneous spring rate of length change in m/s.

Vmax_m = Vmax * rest_length; %convert to meters per second by multiplying by meters per resting length 
% v_relative = muscle_velocity/Vmax_m; %this value was too noisy. Use
% derivative simulink block instead
